simulink model "ESTNavigation"  (R2017a)
settings: Solver=FixedStepAuto  StartTime=0.0  StopTime=2.4  FixedStep=0.01  RelTol=1e-3
settings Model: Creator=xiaodong  LastModifiedBy=xiaodong
settings DataIOCC: SaveFormat=Array  SaveOutput=off  SignalLogging=off  DSMLogging=off  SaveTime=off

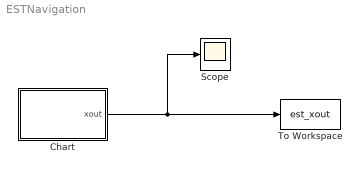
== system ESTNavigation ==
  Chart : Stateflow chart  TreatAsAtomicUnit=on
  Scope : Scope
  To Workspace : ToWorkspace  VariableName=est_xout  SampleTime=-1
  wires:
  Chart/1(xout) -> Scope/1, To Workspace/1

== stateflow chart ESTNavigation/Chart ==
  state M2
    entry:
    A1 = [1.0000  0.0000  0.0099  0.0000;
    0.0000  1.0000  0.0000  0.0099;
    0.0000  0.0000  0.9881  0.0010;
    0.0000  0.0000  0.0010  0.9881];
    Bc1 =[0.0000; 0.0000; 0.0010;-0.0119];
    x = FnM(A1, x) + Bc1;
    xout = x;
    during:
    x = FnM(A1, x) + Bc1;
    xout = x;
  state M3
    entry:
    A3 = [1.0000  0.0000  0.0099  0.0000;
    0.0000  1.0000  0.0000  0.0099;
    0.0000  0.0000  0.9881  0.0010;
    0.0000  0.0000  0.0010  0.9881];
    Bc3 =[0.0000; 0.0000; 0.0091; -0.0091];
    x = FnM(A3, x) + Bc3;
    xout = x;
    during:
    x = FnM(A3, x) + Bc3;
    xout = x;
  state M41
    entry:
    A2 = [1.0000  0.0000  0.0099  0.0000;
    0.0000  1.0000  0.0000  0.0099;
    0.0000  0.0000  0.9881  0.0010;
    0.0000  0.0000  0.0010  0.9881];
    Bc2 =[0.0000; 0.0000; 0.0119; -0.0010];
    x = FnM(A2, x) + Bc2;
    xout = x;
    during:
    x = FnM(A2, x) + Bc2;
    xout = x;
  state M42
    entry:
    A1 = [1.0000  0.0000  0.0099  0.0000;
    0.0000  1.0000  0.0000  0.0099;
    0.0000  0.0000  0.9881  0.0010;
    0.0000  0.0000  0.0010  0.9881];
    Bc1 =[0.0000; 0.0000; 0.0010;-0.0119];
    x = FnM(A1, x) + Bc1;
    xout = x;
    during:
    x = FnM(A1, x) + Bc1;
    xout = x;
  state M43
    during:
    x = [-1;-1;-1;-1];
    xout = x;
  state M1
    entry:
    A2 = [1.0000  0.0000  0.0099  0.0000;
    0.0000  1.0000  0.0000  0.0099;
    0.0000  0.0000  0.9881  0.0010;
    0.0000  0.0000  0.0010  0.9881];
    Bc2 =[0.0000; 0.0000; 0.0119; -0.0010];
    x = FnM(A2, x) + Bc2;
    xout = x;
    during:
    x = FnM(A2, x) + Bc2;
    xout = x;
  state M44
    during:
    x = [-1;-1;-1;-1];
    xout = x;
  M3 -> M1 [order 3] : [0.0083*x(1)-1.0007*x(2)-0.0166*x(3)+ 0.0139*x(4)+ 1>=0]
  (default) -> M1 : {x = [0.4 0.62 0.5 1]';}
  M1 -> M2 [order 1] : [ 0.0049*x(1)-0.9980*x(2)-0.0134*x(3)+ 0.0217*x(4)+ 1<=0]
  M3 -> M41 [order 1] : [-0.0045*x(1)-0.4971*x(2)+ 0.0011*x(3)+ 0.0064*x(4)+ 1<=0]
  M2 -> M3 [order 2] : [-1.0065*x(1)+ 0.0031*x(2)+ 0.0201*x(3)-0.0028*x(4)+ 1<=0]
  M41 -> M42 : [-0.4904*x(1)-0.0049*x(2)+ 0.0030*x(3)+ 1<=0]
  M42 -> M43 : [0.0054*x(1)-0.9710*x(2)-0.0176*x(3)+ 0.0521*x(4)+ 1>=0]
  M2 -> M1 [order 1] : [ 0.0011*x(1)-1.0070*x(2)+ 0.0159*x(3)+ 0.0126*x(4)+1>=0]
  M3 -> M42 [order 2] : [-0.4784*x(1)+ 0.0019*x(2)-0.0449*x(3)+ 0.0168*x(4)+ 1<=0]
  M1 -> M44 [order 2] : [-0.5018*x(1)+ 0.0067*x(3)-0.0030*x(4)+ 1<=0]
  data: u1 function_input; u2 function_input; y function_output; A2 local size=[4,4]; Bc2 local size=[4,1]; x local size=4 =[0.5 0.5 0.5 0.5]'; xout output size=4 =[0.4 0.62 0.5 1]'; A1 local size=[4,4]; A3 local size=[4,4]; Bc1 local size=[4,1]; Bc3 local size=[4,1]
  function y = FnM(u1, u2):
    | function y = FnM(u1, u2)
    | y = u1*u2;
